simulink model "fencerecog"  (R2014b)
settings: Solver=ode45  StartTime=0.0  StopTime=10.0  RelTol=1e-3
libraries: simulink x1
settings Model: Creator=Jackie  LastModifiedBy=Jackie

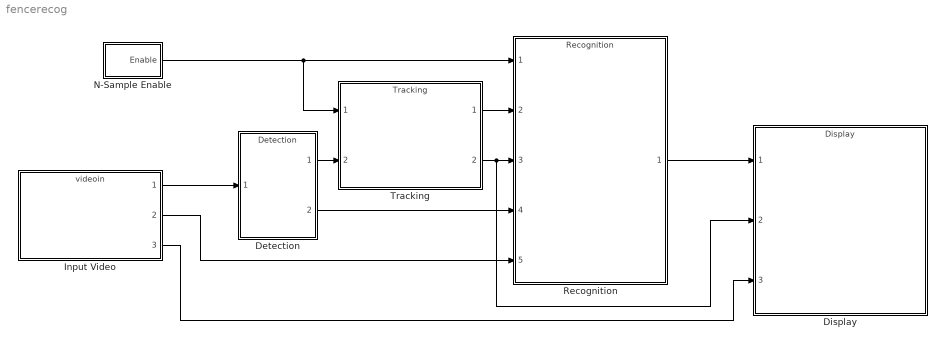
== system fencerecog ==
  Detection : ModelReference  ModelNameDialog=Detection.slx  SimulationMode=Normal  ModelReferenceVersion=1.3  CopyOfModelName=Detection.slx  DefaultDataLogging=on
  Display : ModelReference  ModelNameDialog=Display.slx  SimulationMode=Normal  ModelReferenceVersion=1.5  CopyOfModelName=Display.slx  DefaultDataLogging=on
  Input Video : ModelReference  ModelNameDialog=videoin.slx  SimulationMode=Normal  ModelReferenceVersion=1.3  CopyOfModelName=videoin.slx  DefaultDataLogging=on
  N-Sample Enable : Subsystem  mask{sample=1}
      mask prompts: sample "Trigger Count, N"
  Recognition : ModelReference  ModelNameDialog=Recognition.slx  SimulationMode=Normal  ModelReferenceVersion=1.7  CopyOfModelName=Recognition.slx  DefaultDataLogging=on
  Tracking : ModelReference  ModelNameDialog=Tracking.slx  SimulationMode=Normal  ModelReferenceVersion=1.9  CopyOfModelName=Tracking.slx  DefaultDataLogging=on
  wires:
  Input Video/1 -> Detection/1
  Detection/1 -> Tracking/2
  N-Sample Enable/1(Enable) -> Tracking/1, Recognition/1
  Tracking/2 -> Display/2, Recognition/3
  Tracking/1 -> Recognition/2
  Detection/2 -> Recognition/4
  Recognition/1 -> Display/1
  Input Video/2 -> Recognition/5
  Input Video/3 -> Display/3

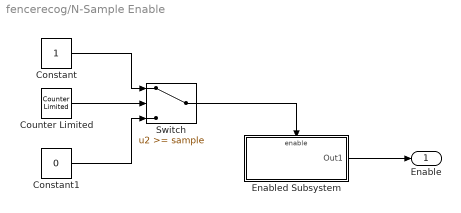
== system fencerecog/N-Sample Enable ==
  Constant : Constant  OutDataTypeStr=boolean
  Constant1 : Constant  Value=0  OutDataTypeStr=boolean
  Counter Limited : simulink/Sources/Counter Limited  uplimit=sample  tsamp=-1
  Enabled Subsystem : Subsystem  TreatAsAtomicUnit=on
  Switch : Switch  Threshold=sample
  Enable : Outport
  wires:
  Counter Limited/1 -> Switch/2
  Constant1/1 -> Switch/3
  Constant/1 -> Switch/1
  Switch/1 -> Enabled Subsystem/Enable
  Enabled Subsystem/1(Out1) -> Enable/1

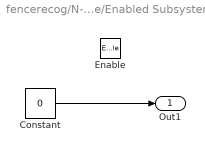
== system fencerecog/N-Sample Enable/Enabled Subsystem ==
  Enable : EnablePort
  Constant : Constant  Value=0  OutDataTypeStr=boolean
  Out1 : Outport  InitialOutput=1
  wires:
  Constant/1 -> Out1/1
